simulink model "scopeInterface_LL"  (R2023b)
settings: Solver=FixedStepAuto  StartTime=0.0  StopTime=30  FixedStep=0.01  RelTol=1e-3
undefined symbols (not defined in the file or in its folder): param
settings Model: PacingRate=1.530000  Creator=Scott.Dahlke  LastModifiedBy=Connor Emmons
settings SolverCC: AlgebraicLoopSolver=TrustRegion
settings DebuggingCC: UnconnectedInputMsg=warning  UnconnectedOutputMsg=warning  UnconnectedLineMsg=warning
settings ModelReferenceCC: EnableRefExpFcnMdlSchedulingChecks=on
settings SFSimCC: CustomCodeUndefinedFunction=UseInterfaceOnly

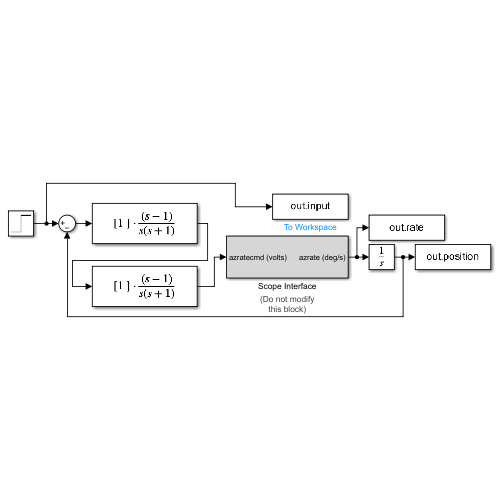
[thumbnail: Simulink's stored preview of the top-level diagram]
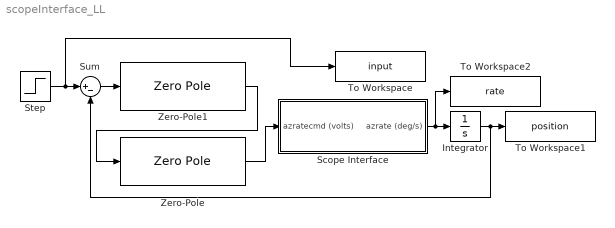
== system scopeInterface_LL ==
  Integrator : Integrator
  Scope Interface : Subsystem
      settings: AttributesFormatString=|
      | (Do not modify
      | this block)
  Step : Step  Time=0  SampleTime=0
  Sum : Sum  Inputs=|+-
  To Workspace : ToWorkspace  VariableName=input  SampleTime=-1
  To Workspace1 : ToWorkspace  VariableName=position  SampleTime=-1
  To Workspace2 : ToWorkspace  VariableName=rate  SampleTime=-1
  Zero-Pole : ZeroPole  Poles=[0 -1]
  Zero-Pole1 : ZeroPole  Poles=[0 -1]
  wires:
  Step/1 -> To Workspace/1, Sum/1
  Zero-Pole/1 -> Scope Interface/1(azratecmd (volts))
  Scope Interface/1(azrate (deg/s)) -> To Workspace2/1, Integrator/1
  Integrator/1 -> Sum/2, To Workspace1/1
  Zero-Pole1/1 -> Zero-Pole/1
  Sum/1 -> Zero-Pole1/1

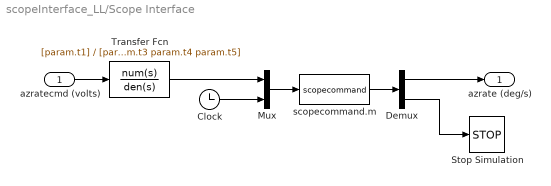
== system scopeInterface_LL/Scope Interface ==
  azratecmd (volts) : Inport
  Clock : Clock
  Demux : Demux  Outputs=2
  Mux : Mux  Inputs=2
  Stop Simulation : Stop
  Transfer Fcn : TransferFcn  Numerator=[param.t1]  Denominator=[param.t3 param.t4 param.t5]
  scopecommand.m : MATLABFcn  MATLABFcn=scopecommand  OutputDimensions=2
  azrate (deg/s) : Outport
  wires:
  azratecmd (volts)/1 -> Transfer Fcn/1
  Mux/1 -> scopecommand.m/1
  Demux/2 -> Stop Simulation/1
  Demux/1 -> azrate (deg/s)/1
  scopecommand.m/1 -> Demux/1
  Transfer Fcn/1 -> Mux/1
  Clock/1 -> Mux/2
